simulink model "Kalman"  (R2023a)
settings: Solver=ode23t  StartTime=0.0  StopTime=1  MaxStep=0.1  RelTol=1e-4
undefined symbols (not defined in the file): Kalman_parameters, State_space
libraries: simulink x2
settings Model: Creator=ПК  LastModifiedBy=ПК

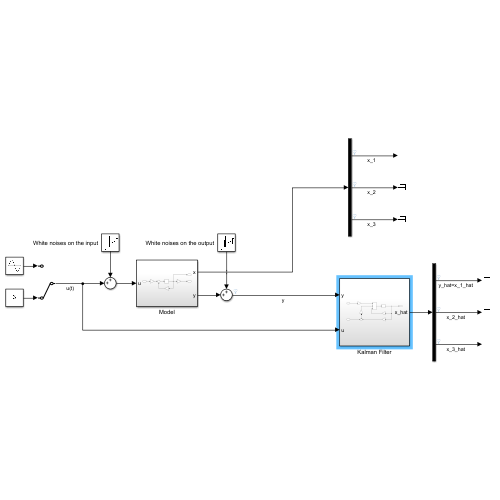
[thumbnail: Simulink's stored preview of the top-level diagram]
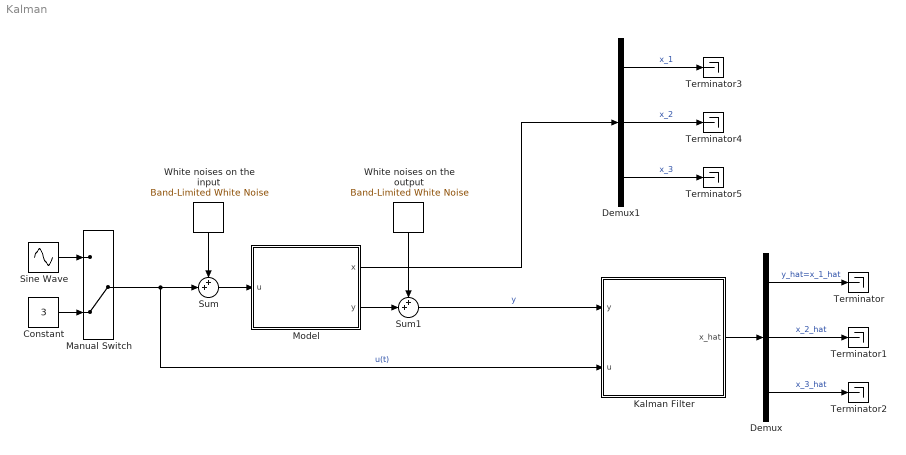
== system Kalman ==
  Constant : Constant  Value=3
  Demux : Demux  Outputs=3
  Demux1 : Demux  Outputs=3
  Kalman Filter : Subsystem
  Manual Switch : ManualSwitch  CurrentSetting=0
  Model : Subsystem
  Sine Wave : Sin  Amplitude=5  Frequency=100  SampleTime=0
  Sum : Sum  Inputs=++|
  Sum1 : Sum  Inputs=++|
  Terminator{,1..5} (6 alike) : Terminator
  White noises on the input : simulink/Sources/Band-Limited White Noise  Cov=[Kalman_parameters.Noise_power_input]  Ts=Kalman_parameters.Ts  seed=[Kalman_parameters.seed_input]
  White noises on the output : simulink/Sources/Band-Limited White Noise  Cov=[Kalman_parameters.Noise_power_output]  Ts=Kalman_parameters.Ts  seed=[Kalman_parameters.seed_output]
  wires:
  Kalman Filter/1(x_hat) -> Demux/1
  Sine Wave/1 -> Manual Switch/1
  Manual Switch/1 -> Kalman Filter/2(u), Sum/2  "u(t)"
  Constant/1 -> Manual Switch/2
  Sum/1 -> Model/1(u)
  White noises on the input/1 -> Sum/1
  White noises on the output/1 -> Sum1/1
  Model/2(y) -> Sum1/2
  Sum1/1 -> Kalman Filter/1(y)  "y"
  Demux/1 -> Terminator/1  "y_hat=x_1_hat"
  Demux/2 -> Terminator1/1  "x_2_hat"
  Demux/3 -> Terminator2/1  "x_3_hat"
  Demux1/3 -> Terminator5/1  "x_3"
  Demux1/1 -> Terminator3/1  "x_1"
  Model/1(x) -> Demux1/1
  Demux1/2 -> Terminator4/1  "x_2"

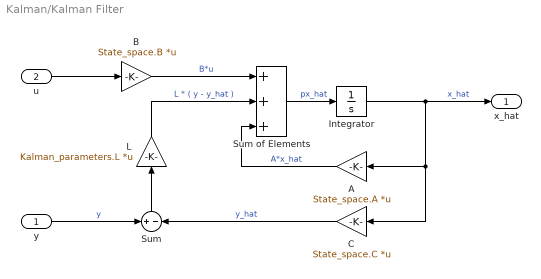
== system Kalman/Kalman Filter ==
  y : Inport
  u : Inport  Port=2
  A : Gain  Gain=State_space.A  Multiplication=Matrix(K*u)
  B : Gain  Gain=State_space.B  Multiplication=Matrix(K*u)
  C : Gain  Gain=State_space.C  Multiplication=Matrix(K*u)
  Integrator : Integrator
  L : Gain  Gain=Kalman_parameters.L  Multiplication=Matrix(K*u)
  Sum : Sum  Inputs=+|-
  Sum of Elements : Sum  Inputs=+++
  x_hat : Outport
  wires:
  B/1 -> Sum of Elements/1  "B*u"
  Sum of Elements/1 -> Integrator/1  "px_hat"
  u/1 -> B/1
  L/1 -> Sum of Elements/2  "L * ( y - y_hat )"
  Integrator/1 -> x_hat/1, A/1, C/1  "x_hat"
  A/1 -> Sum of Elements/3  "A*x_hat"
  Sum/1 -> L/1
  y/1 -> Sum/1  "y"
  C/1 -> Sum/2  "y_hat"

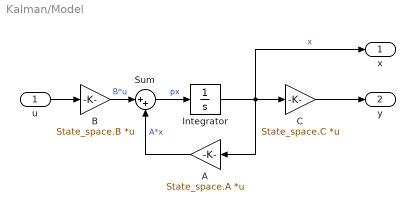
== system Kalman/Model ==
  u : Inport
  A : Gain  Gain=State_space.A  Multiplication=Matrix(K*u)
  B : Gain  Gain=State_space.B  Multiplication=Matrix(K*u)
  Integrator : Integrator
  Sum : Sum  Inputs=|++
  С : Gain  Gain=State_space.C  Multiplication=Matrix(K*u)
  x : Outport
  y : Outport  Port=2
  wires:
  u/1 -> B/1
  B/1 -> Sum/1  "B*u"
  Sum/1 -> Integrator/1  "px"
  A/1 -> Sum/2  "A*x"
  Integrator/1 -> x/1, С/1, A/1  "x"
  С/1 -> y/1
